simulink model "udp_test_model"  (R2020a)
settings: Solver=VariableStepAuto  StartTime=0.0  StopTime=33.0  RelTol=1e-3
PostLoadFcn:
  | if any(exist('dsrtsu_mdlpostloadfcn', 'file') ~= 0), dsrtsu_mdlpostloadfcn('Execute', bdroot); end
InitFcn:
  | , if any(exist('rtifpga_mdlclblib', 'file') ~= 0), rtifpga_mdlclblib('Init', bdroot); end,
libraries: etargetslib x2, rtiethernetlib x2, instrumentlib x1
settings Model: DSRTSU_INTERNAL_RTI_VER=590  DSRTSU_INTERNAL_RTI_TYPE=rti1202  RTICANMMDATA=struct('GeneralSetupData',struct('modelroot','C:\Users\javot\Documents\MATLAB\Bern\simulink','generalsettings',struct('filesettings',struct('destfolder',struct('Name','RTICANMM_FILES','Check',1),'buildfolder',struct('Name','.','Check',1),'AbsDestfolder',struct('Name','C:\Users\javot\Documents\MATLAB\Bern\simulink\RTICANMM_FILES'),'AbsBuildfolder',struct('Name','C:\Users\javot\Documents\MATLAB\Bern\simulink'))),'options',struct('addpaths',1,'rmpaths',1,'addtrcexclusion',true,'cannavigator',struct('checkmonitoring',0),'show_usrtrc',0,'use_usrtrc',0),'advanced',struct('options',ones(1,100)),'MPSetup',{{}},'RTI',struct('Type','GRT','Ver','','Date',''),'modelname','udp_test_model','block','udp_test_model'))  DSRTSU_INTERNAL_RTIFPGA=170  DSRTSU_INTERNAL_RTISTBM_VER=1.4.3  Creator=javot  LastModifiedBy=javot

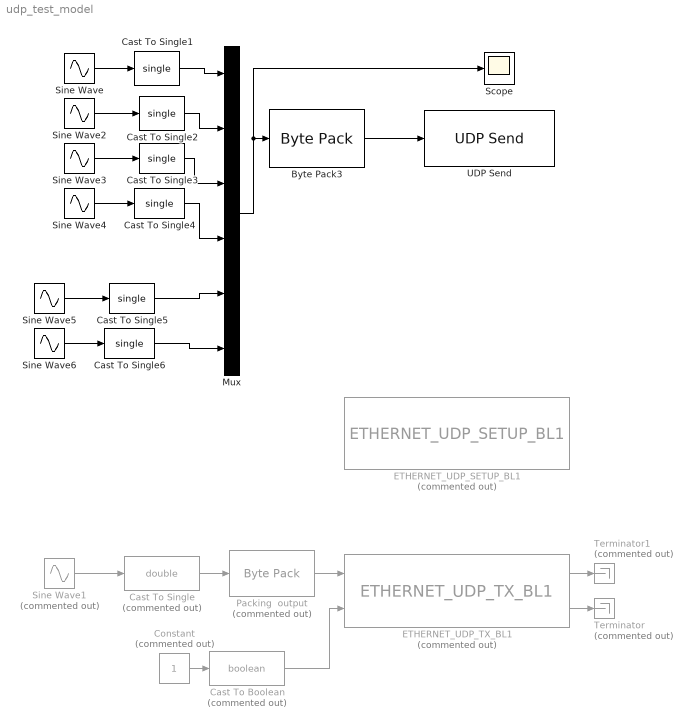
== system udp_test_model ==
  Byte Pack3 : etargetslib/Byte Pack  datatypes={'single'}  byteAlign=1
  Cast To Boolean : DataTypeConversion  Commented=on  OutDataTypeStr=boolean
  Cast To Single : DataTypeConversion  Commented=on  OutDataTypeStr=double
  Cast To Single{1..6} (6 alike) : DataTypeConversion  OutDataTypeStr=single
  Constant : Constant  Commented=on
  ETHERNET_UDP_SETUP_BL1 : rtiethernetlib/ETHERNET_UDP_SETUP_BL1  Commented=on  DSProperties=struct('RTI',struct('Version',uint32(2),'BlockType',struct('isSLSource',uint8(1),'isSLSink',uint8(1),'isHWSource',uint8(0),'isHWSink',uint8(0),'isSetup',uint8(0),'isInline',uint8(1),'isNonInline',uint8(0),'isInterrupt',uint8(0),'isChannelwise',uint8(0)),'IOBoardType','DSETHERNET','UnitType','UDP','Identifier','SETUPUDP','DialogType','ML','BlockSet','RTIETHERNET','SlaveProcessor','NONE'))  RTIBlockInterface=struct('OutputPortsWidth',int32(2),'OutputPortsActive',0,'OutputPortsName',{{['RX Dropped Frames']}},'OutputPortsDataType',{{'SS_DOUBLE'}},'InputPortsWidth',int32([4 1]),'InputPortsActive',int32([0 0]),'InputPortsName',{{['RX Remote IP Filter'],['RX Remote Port Filter']}},'InputPortsDataType',{{'SS_UINT8','SS_UINT16'}},'RWork',{{{'RX_DROPPED_FRAMES',uint32(2)}}},'InitLevel',3,'IconTransparency','on','BlockDisplay',{{['Ethernet UDP/IP\nSetup\n\nSocket ID: 0'],'center'}},'DialogFcn','rtiethernetsetupudpgui','BlockName',struct('Token',{{'ETHERNET_UDP_SETUP_BL1'}}))  RTIBlockParameters=struct('SocketId',{{0,'OFF',[]}},'EnableSocketBind',{{0,'OFF',[0 1]}},'AcceptAnyRxRemoteIp',{{0,'OFF',[0 1]}},'RxRemoteIpNum1',{{'134','OFF',[0 255]}},'RxRemoteIpNum2',{{'105','OFF',[0 255]}},'RxRemoteIpNum3',{{'60','OFF',[0 255]}},'RxRemoteIpNum4',{{'99','OFF',[0 255]}},'EnableDynamicRxRemoteIpFilter',{{0,'OFF',[0 1]}},'AcceptAnyRxRemotePort',{{1,'OFF',[0 1]}},'RxRemotePort',{{'55001','OFF',[1 65535]}},'EnableDynamicRxRemotePortFilter',{{0,'OFF',[0 1]}},'TxRemoteIpNum1',{{'134','OFF',[0 255]}},'TxRemoteIpNum2',{{'105','OFF',[0 255]}},'TxRemoteIpNum3',{{'60','OFF',[0 255]}},'TxRemoteIpNum4',{{'99','OFF',[0 255]}},'TxRemotePort',{{'55001','OFF',[1 65535]}},'SpecifyLocalPort',{{1,'OFF',[0 1]}},'LocalPort',{{'49001','OFF',[1 65535]}},'InterruptMode',{{0,'OFF',[0 1]}},'RxDroppedFramesOutPortMode',{{0,'OFF',[0 1]}},'RemoteIpNumCheck',{{1,'OFF',[0 1]}},'RemotePortCheck',{{0,'OFF',[0 1]}},'LocalPortCheck',{{1,'OFF',[0 1]}},'DHCPserverModeEnabled',{{0,'OFF',[0 1]}},'TLCFileName',{{'rtiethernetsetupudp','OFF',[]}})  RTISFcnParameters=struct('SocketId','double','EnableSocketBind','int32','AcceptAnyRxRemoteIp','int32','RxRemoteIpNum1','uint8','RxRemoteIpNum2','uint8','RxRemoteIpNum3','uint8','RxRemoteIpNum4','uint8','EnableDynamicRxRemoteIpFilter','int32','AcceptAnyRxRemotePort','int32','RxRemotePort','uint16','EnableDynamicRxRemotePortFilter','int32','TxRemoteIpNum1','uint8','TxRemoteIpNum2','uint8','TxRemoteIpNum3','uint8','TxRemoteIpNum4','uint8','TxRemotePort','uint16','SpecifyLocalPort','int32','LocalPort','uint16','InterruptMode','int32','RxDroppedFramesOutPortMode','int32','DHCPserverModeEnabled','int32','TLCFileName','char')  RTIBlockParaDefault=struct('SocketId',-1,'EnableSocketBind',1,'AcceptAnyRxRemoteIp',1,'RxRemoteIpNum1',0,'RxRemoteIpNum2',0,'RxRemoteIpNum3',0,'RxRemoteIpNum4',0,'EnableDynamicRxRemoteIpFilter',0,'AcceptAnyRxRemotePort',1,'RxRemotePort',49002,'EnableDynamicRxRemotePortFilter',0,'TxRemoteIpNum1',0,'TxRemoteIpNum2',0,'TxRemoteIpNum3',0,'TxRemoteIpNum4',0,'TxRemotePort',49002,'SpecifyLocalPort',0,'LocalPort',49001,'InterruptMode',0,'RxDroppedFramesOutPortMode',0,'RemoteIpNumCheck',0,'RemotePortCheck',0,'LocalPortCheck',0,'DHCPserverModeEnabled',0,'TLCFileName','rtiethernetsetupudp')
      settings: SourceProductName=dSPACE RTI Ethernet Blockset
  ETHERNET_UDP_TX_BL1 : rtiethernetlib/ETHERNET_UDP_TX_BL1  Commented=on  DSProperties=struct('RTI',struct('Version',uint32(1),'BlockType',struct('isSLSource',uint8(1),'isSLSink',uint8(1),'isHWSource',uint8(0),'isHWSink',uint8(1),'isSetup',uint8(0),'isInline',uint8(1),'isNonInline',uint8(0),'isInterrupt',uint8(0),'isChannelwise',uint8(0)),'IOBoardType','DSETHERNET','UnitType','UDP','Identifier','TXUDP','DialogType','ML','BlockSet','RTIETHERNET','SlaveProcessor','NONE'))  RTIBlockInterface=struct('OutputPortsWidth',int32([1 1]),'OutputPortsActive',[1 1],'OutputPortsName',{{'Status',['Sent Frames']}},'OutputPortsDataType',{{'SS_UINT32','SS_DOUBLE'}},'InputPortsWidth',int32([8 1 1 4 1]),'InputPortsActive',[1 1 0 0 0],'InputPortsName',{{'Data','Enable',['Bytes to Send'],['Remote IP'],['Remote Port']}},'InputPortsDataType',{{'SS_UINT8','SS_BOOLEAN','SS_UINT32','SS_UINT8','SS_UINT16'}},'RWork',{{{'SENT_FRAMES',uint32(1)}}},'InitLevel',3,'IconTransparency','on','BlockDisplay',{{['Ethernet UDP/IP\nTX\n\nSocket ID: 0'],'center'}},'DialogFcn','rtiethernettxudpgui','BlockName',struct('Token',{{'ETHERNET_UDP_TX_BL1'}}))  RTIBlockParameters=struct('SocketIdIndex',{{2,'OFF',[1 2]}},'SocketId',{{0,'OFF',[-1 inf]}},'RemoteIp',{{'134.105.60.99','OFF',[]}},'RemotePort',{{55001,'OFF',[]}},'LocalPort',{{49001,'OFF',[]}},'EnableDynamicRemoteIp',{{0,'OFF',[0 1]}},'EnableDynamicRemotePort',{{0,'OFF',[0 1]}},'FrameSize',{{'8','OFF',[1 65507]}},'EnableVariableFrameSize',{{0,'OFF',[0 1]}},'SentFramesOutPortMode',{{1,'OFF',[0 1]}},'RemoteIpNum',{{[134 105 60 99],'OFF',[0 255]}},'RemotePortNum',{{55001,'OFF',[0 65535]}},'TLCFileName',{{'rtiethernettxudp','OFF',[]}})  RTISFcnParameters=struct('SocketIdIndex','int32','SocketId','double','EnableDynamicRemoteIp','int32','EnableDynamicRemotePort','int32','FrameSize','uint16','EnableVariableFrameSize','int32','SentFramesOutPortMode','int32','RemoteIpNum','uint8','RemotePortNum','uint16','TLCFileName','char')  RTIBlockParaDefault=struct('SocketIdIndex',1,'SocketId',-1,'RemoteIp',['<NOT AVAILABLE>'],'RemotePort',['<NOT AVAILABLE>'],'LocalPort',['<NOT AVAILABLE>'],'EnableDynamicRemoteIp',0,'EnableDynamicRemotePort',0,'FrameSize',1024,'EnableVariableFrameSize',0,'SentFramesOutPortMode',1,'RemoteIpNum',[0 0 0 0],'RemotePortNum',0,'TLCFileName','rtiethernettxudp')
      settings: SourceProductName=dSPACE RTI Ethernet Blockset
  Mux : Mux  Inputs=6
  Packing  output : etargetslib/Byte Pack  Commented=on  datatypes={'double'}  byteAlign=1
  Scope : Scope
  Sine Wave : Sin  Amplitude=0.25  Frequency=10  SampleTime=0.001
  Sine Wave1 : Sin  Commented=on  SampleTime=0.001
  Sine Wave2 : Sin  Amplitude=0.5  Frequency=2  SampleTime=0.001
  Sine Wave3 : Sin  Frequency=5  SampleTime=0.001
  Sine Wave4 : Sin  Amplitude=1.25  Frequency=0.8  SampleTime=0.001
  Sine Wave5 : Sin  Amplitude=10  Frequency=5  SampleTime=0.001
  Sine Wave6 : Sin  Amplitude=5  Frequency=0.8  SampleTime=0.001
  Terminator : Terminator  Commented=on
  Terminator1 : Terminator  Commented=on
  UDP Send : instrumentlib/UDP Send  Host=134.105.60.99  Port=55001  LocalPort=-1  EnablePortSharing=off  ByteOrder=BigEndian  OutputDatagramPacketSize=512  EnableBlockingMode=on  LocalAddress=0.0.0.0
  wires:
  ETHERNET_UDP_TX_BL1/1 -> Terminator1/1
  Sine Wave1/1 -> Cast To Single/1
  ETHERNET_UDP_TX_BL1/2 -> Terminator/1
  Constant/1 -> Cast To Boolean/1
  Cast To Boolean/1 -> ETHERNET_UDP_TX_BL1/2
  Cast To Single/1 -> Packing  output/1
  Packing  output/1 -> ETHERNET_UDP_TX_BL1/1
  Mux/1 -> Scope/1, Byte Pack3/1
  Byte Pack3/1 -> UDP Send/1
  Cast To Single1/1 -> Mux/1
  Sine Wave/1 -> Cast To Single1/1
  Sine Wave2/1 -> Cast To Single2/1
  Cast To Single2/1 -> Mux/2
  Cast To Single3/1 -> Mux/3
  Sine Wave3/1 -> Cast To Single3/1
  Sine Wave4/1 -> Cast To Single4/1
  Cast To Single4/1 -> Mux/4
  Cast To Single6/1 -> Mux/6
  Sine Wave6/1 -> Cast To Single6/1
  Cast To Single5/1 -> Mux/5
  Sine Wave5/1 -> Cast To Single5/1
